simulink model "ASMC2000_2021a_2604"  (R2021a)
settings: Solver=VariableStepAuto  StartTime=0.0  StopTime=20  FixedStep=0.001  RelTol=1e-3
settings Model: Creator=ADMIN  LastModifiedBy=pc
settings DebuggingCC: UnderSpecifiedDimensionMsg=warning

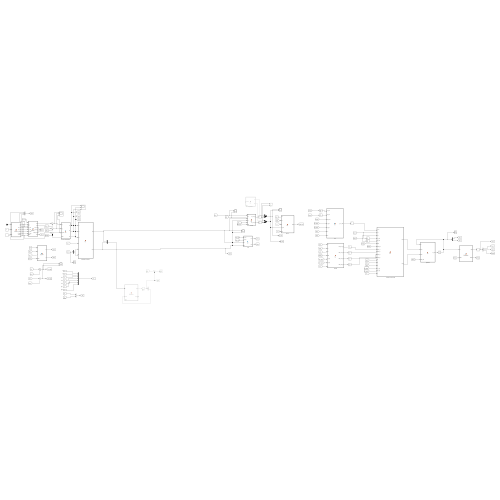
[thumbnail: Simulink's stored preview of the top-level diagram]
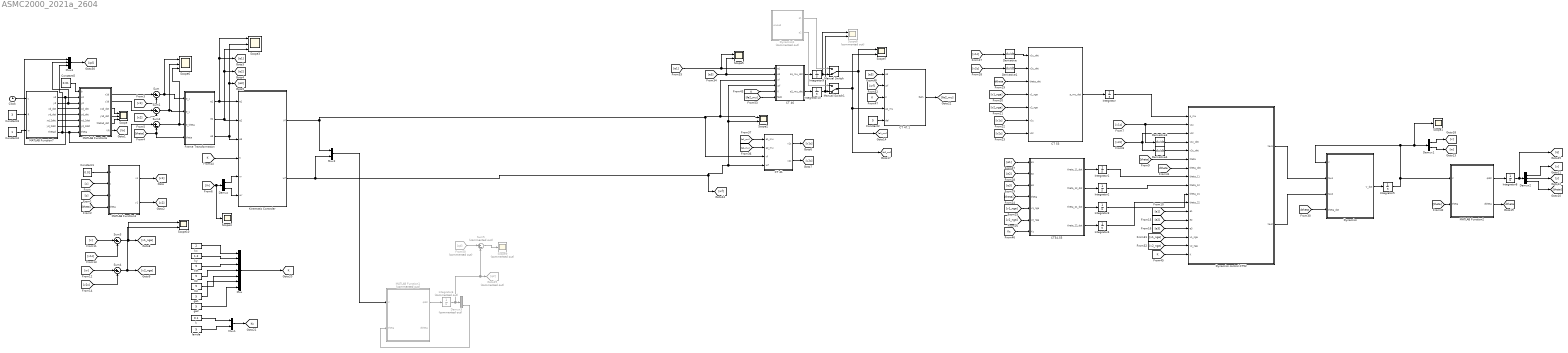
== system ASMC2000_2021a_2604 ==
  CT 41 : MATLAB Function  TreatAsAtomicUnit=on
  CT 46 : MATLAB Function  TreatAsAtomicUnit=on
  CT 47.1 : MATLAB Function  TreatAsAtomicUnit=on
  CT 53 : MATLAB Function  TreatAsAtomicUnit=on
  CT54,55 : MATLAB Function  TreatAsAtomicUnit=on
  Clock : Clock
  Constant1 : Constant  Value=0.01
  Constant2 : Constant  Value=5
  Constant3 : Constant  Value=3
  Constant4 : Constant
  Constant5 : Constant  Value=0.01
  Demux : Demux  Outputs=2
  Demux1 : Demux  Outputs=2
  Demux2 : Demux  Outputs=3
  Demux3 : Demux  Commented=on  Outputs=3
  Derivative{,1,3..4} (4 alike) : Derivative
  Dynamics : MATLAB Function  TreatAsAtomicUnit=on
  Dynamics control.CT52 : MATLAB Function  TreatAsAtomicUnit=on
  Dynamics1 : MATLAB Function  Commented=on  TreatAsAtomicUnit=on
  Frame Transformation : MATLAB Function  TreatAsAtomicUnit=on
  From50 : From  Commented=on  GotoTag=qd
  Goto29 : Goto  Commented=on  GotoTag=q2
  Integrator : Integrator  InitialCondition=[0;0;0]
  Integrator{1..4,9..10} (6 alike) : Integrator
  Integrator5 : Integrator  InitialCondition=[0;0]
  Integrator6 : Integrator  Commented=on  InitialCondition=[0;0;0]
  Integrator8 : Integrator  InitialCondition=[0;0;0]
  K2 : Constant  Value=5
  Kd : Constant  Value=5
  Kinematic Controler : MATLAB Function  TreatAsAtomicUnit=on
  MATLAB Function1 : MATLAB Function  Commented=on  TreatAsAtomicUnit=on
  MATLAB Function2 : MATLAB Function  TreatAsAtomicUnit=on
  MATLAB Function3 : MATLAB Function  TreatAsAtomicUnit=on
  MATLAB Function6 : MATLAB Function  TreatAsAtomicUnit=on
  MATLAB Function7 : MATLAB Function  TreatAsAtomicUnit=on
  Manual Switch : ManualSwitch  CurrentSetting=0
  Manual Switch1 : ManualSwitch  CurrentSetting=0
  Mux : Mux  Inputs=7
  Mux1 : Mux  Inputs=2
  Mux2 : Mux  Inputs=2
  Mux3 : Mux  Inputs=3
  Scope : Scope  NumInputPorts=3
  Scope1 : Scope
  Scope{2,5,7,10} (4 alike) : Scope  NumInputPorts=2
  Scope3 : Scope  NumInputPorts=3
  Scope4 : Scope
  Scope6 : Scope  NumInputPorts=3
  Scope8 : Scope  Commented=on  NumInputPorts=2
  Scope9 : Scope  Commented=on
  Sum{,1..4} (5 alike) : Sum  Inputs=|+-
  Sum5 : Sum  Commented=on  Inputs=|+-
  ga1 : Constant  Value=5
  ga2 : Constant  Value=5
  k : Constant  Value=0.1
  kth : Constant  Value=5
  kx : Constant  Value=2
  ky : Constant  Value=1.2
  lamda : Constant  Value=5
  tag scope: K=global, Kc=global, dtheta=global
  wires:
  MATLAB Function7/2(yd) -> Mux3/2, MATLAB Function6/3(yd)
  MATLAB Function6/2(y1d) -> Sum1/1
  MATLAB Function7/7(thetad) -> Mux3/3, Sum2/1, MATLAB Function6/8(theta)
  MATLAB Function7/6(yd_2dot) -> MATLAB Function6/7(yd_2dot)
  MATLAB Function7/3(xd_dot) -> MATLAB Function6/4(xd_dot)
  MATLAB Function6/1(x1d) -> Sum/1
  Clock/1 -> MATLAB Function7/1(t)
  MATLAB Function7/1(xd) -> Mux3/1, MATLAB Function6/2(xd)
  Constant5/1 -> MATLAB Function6/1(b)
  MATLAB Function7/5(xd_2dot) -> MATLAB Function6/6(xd_2dot)
  MATLAB Function7/4(yd_dot) -> MATLAB Function6/5(yd_dot)
  Sum/1 -> Scope6/1, Frame Transformation/1(e_x)
  Sum1/1 -> Scope6/2, Frame Transformation/2(e_y)
  Constant1/1 -> MATLAB Function3/1(b)
  [y] -> MATLAB Function3/3(y)
  [x] -> MATLAB Function3/2(x)
  [theta] -> MATLAB Function3/4(theta)
  MATLAB Function3/1(x1) -> [x1]
  [x1] -> Sum/2
  [theta] -> Sum2/2, Frame Transformation/4(theta)
  MATLAB Function3/2(y1) -> [x2]
  [x2] -> Sum1/2
  Sum2/1 -> Scope6/3, Frame Transformation/3(e_theta)
  Frame Transformation/2(e2) -> Scope3/3, [e2], Kinematic Controler/2(e2)
  Frame Transformation/3(e3) -> [e3], Scope3/2, Kinematic Controler/3(e3)
  MATLAB Function6/6(VR) -> [Vr]
  [Vr] -> Scope4/1, Demux/1
  Demux/1 -> Kinematic Controler/5(vr)
  Demux/2 -> Kinematic Controler/6(wr)
  Frame Transformation/1(e1) -> Scope3/1, [e1], Kinematic Controler/1(e1)
  CT 41/1(v1c) -> [v1c]
  CT 41/2(v2c) -> [v2c]
  [v] -> Sum3/1
  [v1c] -> Sum3/2
  [w] -> Sum4/1
  [v2c] -> Sum4/2
  Sum3/1 -> Scope10/1, [v1_nga]
  Sum4/1 -> Scope10/2, [v2_nga]
  [v1c] -> Derivative/1
  Derivative/1 -> CT 53/1(v1c_dot)
  [v2c] -> Derivative1/1
  Derivative1/1 -> CT 53/2(v2c_dot)
  [dtheta] -> CT 53/3(theta_dot)
  [v1_nga] -> CT 53/4(v1_nga)
  [v2_nga] -> CT 53/5(v2_nga)
  CT 53/1(p_mu_dot) -> Integrator/1
  Integrator/1 -> Dynamics control.CT52/1(p_mu)
  [v1c] -> CT 53/6(v1c)
  [v2_nga] -> CT54,55/6(v2_nga)
  [e1] -> CT54,55/1(e1)
  [e2] -> CT54,55/2(e2)
  [e3] -> CT54,55/3(e3)
  [theta] -> CT54,55/4(theta)
  [v1_nga] -> CT54,55/5(v1_nga)
  CT54,55/1(theta_11_dot) -> Integrator1/1
  CT54,55/2(theta_12_dot) -> Integrator2/1
  CT54,55/3(theta_21_dot) -> Integrator3/1
  CT54,55/4(theta_22_dot) -> Integrator4/1
  Integrator1/1 -> Dynamics control.CT52/8(theta_11)
  Integrator2/1 -> Dynamics control.CT52/9(theta_12)
  Integrator3/1 -> Dynamics control.CT52/10(theta_21)
  Integrator4/1 -> Dynamics control.CT52/11(theta_22)
  [v1c] -> Derivative3/1, Dynamics control.CT52/2(v1c)
  [v2c] -> Dynamics control.CT52/3(v2c), Derivative4/1
  Derivative3/1 -> Dynamics control.CT52/4(v1c_dot)
  Derivative4/1 -> Dynamics control.CT52/5(v2c_dot)
  [theta] -> Dynamics control.CT52/6(theta)
  [e1] -> Dynamics control.CT52/12(e1)
  [e2] -> Dynamics control.CT52/13(e2)
  [e3] -> Dynamics control.CT52/14(e3)
  [dtheta] -> Dynamics/4(theta_dot)
  Dynamics/1(V_dot) -> Integrator5/1
  Integrator5/1 -> MATLAB Function2/1(V), Dynamics/1(V), Scope1/1, Demux1/1
  Demux1/2 -> [w]
  MATLAB Function2/1(qdot) -> Integrator8/1
  Demux2/1 -> [x]
  [v2c] -> CT 53/7(v2c)
  [v1_nga] -> Dynamics control.CT52/15(v1_nga)
  [v2_nga] -> Dynamics control.CT52/16(v2_nga)
  MATLAB Function6/3(x1d_dot) -> Scope/1
  MATLAB Function6/4(y1d_dot) -> Scope/2
  MATLAB Function6/5(thetad_dot) -> Scope/3
  Kinematic Controler/1(Vf) -> Mux2/1, Scope2/1, CT 46/3(vf), CT 41/3(vf)
  [e1] -> CT 46/1(e1), Scope5/1
  [e3] -> Scope5/2, CT 46/2(e3)
  CT 46/1(a1_mu_dot) -> Integrator9/1
  CT 46/2(a2_mu_dot) -> Integrator10/1
  Manual Switch/1 -> [a1_mu], Scope7/1
  [a2_mu] -> CT 41/2(a2_mu)
  [a1_mu] -> CT 41/1(a1_mu)
  Demux1/1 -> [v]
  [dtheta] -> Dynamics control.CT52/7(theta_dot)
  [theta] -> MATLAB Function2/2(theta)
  Integrator8/1 -> [q], Demux2/1
  Demux2/2 -> [y]
  Demux2/3 -> [theta]
  MATLAB Function2/2(dtheta) -> [dtheta]
  Dynamics control.CT52/1(tau1) -> Dynamics/2(tau1)
  Dynamics control.CT52/2(tau2) -> Dynamics/3(tau2)
  Mux/1 -> [K]
  kx/1 -> Mux/1
  ky/1 -> Mux/2
  kth/1 -> Mux/3
  K2/1 -> Mux/4
  Kd/1 -> Mux/5
  ga1/1 -> Mux/6
  ga2/1 -> Mux/7
  [K] -> CT 46/5(K)
  [K] -> Kinematic Controler/4(K)
  [K] -> Dynamics control.CT52/17(K)
  Mux1/1 -> [Kc]
  k/1 -> Mux1/1
  lamda/1 -> Mux1/2
  [Kc] -> CT54,55/7(Kc)
  Manual Switch1/1 -> CT 47.1/4(a2_mu), [a2_mu], Scope7/2
  [e3] -> CT 47.1/1(e3)
  [K] -> CT 47.1/3(K)
  [wf] -> CT 47.1/2(wf)
  CT 47.1/1(fa2h) -> [fa2_mu]
  Kinematic Controler/2(wf) -> Mux2/2, CT 46/4(wf), Scope2/2, CT 41/4(wf), [wf]
  Constant2/1 -> CT 47.1/5(del)
  Constant3/1 -> MATLAB Function7/2(R)
  Constant4/1 -> MATLAB Function7/3(w)
  [fa2_mu] -> CT 46/6(fa2h)
  Integrator10/1 -> Scope8/2, Manual Switch1/2
  Integrator9/1 -> Scope8/1, Manual Switch/2
  Dynamics1/1(a1) -> Manual Switch/1
  Dynamics1/2(a2) -> Manual Switch1/1
  Integrator6/1 -> Demux3/1, Sum5/2, Goto29/1
  MATLAB Function1/1(qdot) -> Integrator6/1
  Mux2/1 -> MATLAB Function1/1(V)
  Mux3/1 -> [qd]
  From50/1 -> Sum5/1
  Sum5/1 -> Scope9/1
  Demux3/3 -> MATLAB Function1/2(theta)

== matlab function ASMC2000_2021a_2604/Dynamics control.CT52 ==
  data: p_mu input; v1c input; v2c input; v1c_dot input; v2c_dot input; theta input; theta_dot input; theta_11 input; theta_12 input; theta_21 input; theta_22 input; e1 input; tau1 output; e2 input; e3 input; v1_nga input; v2_nga input; tau2 output; K input
function [tau1,tau2]  = fcn(p_mu,v1c,v2c,v1c_dot,v2c_dot,theta,theta_dot,theta_11,theta_12,theta_21,theta_22,e1,e2,e3,v1_nga,v2_nga,K)

% kd=0.01;
% K2=5;
kd=K(5);
K2=K(4);
A=[v1_nga; v2_nga];%2x1
B=[v1c_dot  v2c_dot  theta_dot*v2c;...
    v2c_dot  v1c_dot  -theta_dot*v1c]; %2x3

V1_x=-e1*cos(theta)+e2*sin(theta);
V1_y=-e1*sin(theta)-e2*cos(theta);
V1_theta=-sin(e3)/K2;

C=[theta_11*(V1_x*cos(theta)+V1_y*sin(theta))+theta_12*V1_theta;...
    theta_21*(V1_x*cos(theta)+V1_y*sin(theta))-theta_22*V1_theta];

tau=-kd*A+B*p_mu-C;
tau1=tau(1);tau2=tau(2);

%công thức 52

== matlab function ASMC2000_2021a_2604/CT 53 ==
  data: v1c_dot input; p_mu_dot output; v2c_dot input; theta_dot input; v1_nga input; v2_nga input; v1c input; v2c input
function p_mu_dot  = fcn(v1c_dot,v2c_dot,theta_dot,v1_nga,v2_nga,v1c,v2c)

gamma=5;

A=[v1c_dot v2c_dot; v2c_dot v1c_dot; theta_dot*v2c -theta_dot*v1c];
B=[v1_nga; v2_nga];
p_mu_dot=-gamma*A*B;

%công thức 53;

== matlab function ASMC2000_2021a_2604/Dynamics ==
  data: V input; V_dot output; tau1 input; tau2 input; theta_dot input
function V_dot  = fcn(V,tau1,tau2,theta_dot)
r=0.15;
b=0.75;
Ic=15.625;
Iw=0.005;
Im=0.0025;
mw=1;
mc=30;
d=0.3;
I=mc*d^2+2*mw*b^2+Ic+2*Im;
m=mc+2*mw;

M=[(r^2/(4*b^2))*(m*b^2+I)+Iw    (r^2/(4*b^2))*(m*b^2-I);...
    (r^2/(4*b^2))*(m*b^2-I)    (r^2/(4*b^2))*(m*b^2+I)+Iw];
C=[0   (r^2/(2*b))*(mc*d*theta_dot);...
    -(r^2/(2*b))*(mc*d*theta_dot)   0];
B=[1 0;0 1];
tau=[tau1;tau2];
V_dot=M\(B*tau-C*V);
%công thức 27

== matlab function ASMC2000_2021a_2604/MATLAB Function7 ==
  data: t input; xd output; yd output; xd_dot output; yd_dot output; xd_2dot output; yd_2dot output; thetad output; R input; w input
function [xd,yd,xd_dot,yd_dot,xd_2dot,yd_2dot,thetad] = quydao(t,R,w)
%% Khoi tao quy dao chuyen dong
%R=5; %ban kinh quy dao
%w=0.8; %rad/s =2*pi*f f=w/2/pi -> T=1/f
xd=R*cos(w*t);
yd=R*sin(w*t);
xd_dot=-R*w*sin(w*t);
yd_dot=R*w*cos(w*t);
x0d_dot=-R*w*sin(w);
y0d_dot=R*w*cos(w);
xd_2dot=-R*w^2*cos(w*t);
yd_2dot=-R*w^2*sin(w*t);
theta0=atan2(y0d_dot,x0d_dot)-w;
thetad=w*t + theta0;

== matlab function ASMC2000_2021a_2604/Dynamics1 ==
  data: unused input; a1 output; a2 output
function [a1,a2]  = fcn(~)
r=0.15;
b=0.75;
a1=1/r;
a2=b/r;

== matlab function ASMC2000_2021a_2604/MATLAB Function2 ==
  data: V input; qdot output; theta input; dtheta output
function [qdot,dtheta]=Kinematics(V,theta)

S=[cos(theta) 0; sin(theta) 0; 0 1];
qdot=S*V;
dtheta=qdot(3);

%ct37

== matlab function ASMC2000_2021a_2604/CT 46 ==
  data: e1 input; a1_mu_dot output; e3 input; a2_mu_dot output; vf input; wf input; K input; fa2h input
function [a1_mu_dot,a2_mu_dot] = fcn(e1,e3,vf,wf,K,fa2h)
K2=K(5);
gamma1=K(6);gamma2=K(7);
%%
a1_mu_dot=gamma1*e1*vf;
% f0a2=gamma2*wf*sin(e3)/K2; %47.2
a2_mu_dot=(gamma2*wf*sin(e3)/K2)+fa2h; %46
%ct46

== matlab function ASMC2000_2021a_2604/CT 47.1 ==
  data: e3 input; wf input; K input; fa2h output; a2_mu input; del input
function fa2h = fcn(e3,wf,K,a2_mu,del)
K2=K(5);
gamma2=K(7);

f0a2=gamma2*((wf*sin(e3))/K2); %46

if a2_mu>del
    fa2h=0;
else 
    fa2h=(1-a2_mu/del)^2*(f0a2^2+1);
end

== matlab function ASMC2000_2021a_2604/MATLAB Function1 ==
  data: V input; qdot output; theta input; dtheta output
function [qdot,dtheta]=Kinematics(V,theta)

S=[cos(theta) 0; sin(theta) 0; 0 1];
qdot=S*V;
dtheta=qdot(3);

%ct37

== matlab function ASMC2000_2021a_2604/Frame Transformation ==
  data: e_x input; e1 output; e_y input; e_theta input; e2 output; e3 output; theta input
function [e1,e2,e3] = fcn(e_x,e_y,e_theta,theta)
A=[cos(theta) sin(theta) 0;-sin(theta) cos(theta) 0;0 0 1];
B=[e_x;e_y;e_theta];
C=A*B;
e1=C(1);
e2=C(2);
e3=C(3);
% công thức 34

== matlab function ASMC2000_2021a_2604/Kinematic Controler ==
  data: e1 input; Vf output; e2 input; e3 input; K input; wf output; vr input; wr input
function [Vf,wf] = fcn(e1,e2,e3,K,vr,wr)
K1=K(1);K2=K(2);K3=K(3);
Vf=vr*cos(e3)+ K1*e1;
wf=wr+vr*K2*e2 + K3*sin(e3);

%công thức 35

== matlab function ASMC2000_2021a_2604/MATLAB Function3 ==
  data: b input; x1 output; y1 output; x input; y input; theta input
function [x1,y1] = quydao(b,x,y,theta)
%% Thiet lap quy dao chuyen dong cho robot
%theta=atan2(yd_dot,xd_dot);
x1=x+b*cos(theta);
y1=y+b*sin(theta);

== matlab function ASMC2000_2021a_2604/CT54,55 ==
  data: e1 input; theta_11_dot output; e2 input; e3 input; theta input; v1_nga input; v2_nga input; theta_12_dot output; theta_21_dot output; theta_22_dot output; Kc input
function [theta_11_dot,theta_12_dot,theta_21_dot,theta_22_dot] = fcn(e1,e2,e3,theta,v1_nga,v2_nga,Kc)

K2=Kc(1);
lamda=Kc(2);


V1_x=-e1*cos(theta)+e2*sin(theta);
V1_y=-e1*sin(theta)-e2*cos(theta);
V1_theta=-sin(e3)/K2;

theta_11_dot=lamda*(V1_x*cos(theta)+V1_y*sin(theta))*v1_nga;
theta_12_dot=lamda*V1_theta*v1_nga;

theta_21_dot=lamda*(V1_x*cos(theta)+V1_y*sin(theta))*v2_nga;
theta_22_dot=lamda*(-V1_theta)*v2_nga;

%công thức 54,55

== matlab function ASMC2000_2021a_2604/CT 41 ==
  data: a1_mu input; v1c output; a2_mu input; v2c output; vf input; wf input
function [v1c,v2c] = fcn(a1_mu,a2_mu,vf,wf)

A=[a1_mu a2_mu;a1_mu -a2_mu];
B=[vf;wf];

V=A*B;
v1c=V(1);
v2c=V(2);
%ct 41

== matlab function ASMC2000_2021a_2604/MATLAB Function6 ==
  data: b input; x1d output; y1d output; x1d_dot output; y1d_dot output; thetad_dot output; xd input; yd input; xd_dot input; yd_dot input; xd_2dot input; yd_2dot input; theta input; VR output
function [x1d,y1d,x1d_dot,y1d_dot,thetad_dot,VR] = quydao(b,xd,yd,xd_dot,yd_dot,xd_2dot,yd_2dot,theta)
%% Thiet lap quy dao chuyen dong cho robot
%theta=atan2(yd_dot,xd_dot);
x1d=xd+b*cos(theta);
y1d=yd+b*sin(theta);
wd=(yd_2dot*xd_dot - xd_2dot*yd_dot)/(xd_dot^2+yd_dot^2);
x1d_dot=xd_dot-b*wd*sin(theta);
y1d_dot=yd_dot+b*wd*cos(theta);
thetad_dot=wd;
rot=[cos(theta) 0; sin(theta) 0; 0 1];
p_dot=[xd_dot; yd_dot; wd];
VR=rot\p_dot;
